simulink model "automata_learning"  (R2022a)
settings: Solver=FixedStepAuto  StartTime=0.0  StopTime=10.0  FixedStep=0.01  RelTol=1e-3
settings Model: Creator=diego  LastModifiedBy=diego

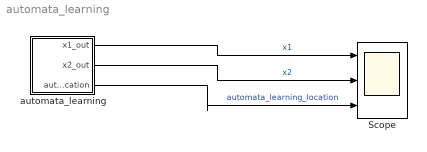
== system automata_learning ==
  Scope : Scope  NumInputPorts=3
  automata_learning : Stateflow chart  TreatAsAtomicUnit=on
  wires:
  automata_learning/1(x1_out) -> Scope/1  "x1"
  automata_learning/2(x2_out) -> Scope/2  "x2"
  automata_learning/3(automata_learning_location) -> Scope/3  "automata_learning_location"

== stateflow chart automata_learning/automata_learning ==
  settings: updateMethod=CONTINUOUS
  state loc1
    du:
    x1_dot = 17709872814793.0 * x2 / 147573952589676410000.0 - 4885549301075.0 * x1 / 295147905179352830000.0 - 25560522869469.0 * x1 * x2 / 36893488147419103000.0 + 23348987725423.0 * x1 ^ 2.0 / 295147905179352830000.0 + 37317396741413.0 * x2 ^ 2.0 / 36893488147419103000.0 + 0.9999999961747696;
    x2_dot = 4503599648254823.0 * x1 / 4503599627370496.0 + 475678987389.0 * x2 / 9223372036854776000.0 - 192670781808847.0 * x1 * x2 / 295147905179352830000.0 + 55569792035993.0 * x1 ^ 2.0 / 1180591620717411300000.0 + 336092630055397.0 * x2 ^ 2.0 / 295147905179352830000.0 - 0.0000000020426695939894023;
    x1_out=x1;
    x2_out=x2;
    automata_learning_location =1;
  state loc2
    du:
    x1_dot = 11278941379.0 * x1 * x2 / 2251799813685248.0 - 614502682225.0 * x2 / 36028797018963968.0 - 1617979564213.0 * x1 / 144115188075855872.0 + 2104648728409.0 * x1 ^ 2.0 / 1152921504606846980.0 - 9007161403513265.0 * x2 ^ 2.0 / 9007199254740992.0 + 0.00001782211096618136;
    x2_dot = 2069062415.0 * x1 / 1125899906842624.0 + 14700152253.0 * x2 / 4503599627370496.0 - 238660367459.0 * x1 * x2 / 288230376151711740.0 - 399866766279.0 * x1 ^ 2.0 / 1152921504606846980.0 - 55380855441.0 * x2 ^ 2.0 / 72057594037927936.0 - 1.0000030969954306;
    x1_out=x1;
    x2_out=x2;
    automata_learning_location =2;
  loc1 -> loc2 : [0.0009391 * x2 - 0.4996 * x1 + 1.0 < 0.0]
  (default) -> loc1 : {x1 = 0.0;
      | x2 = 0.0;}
  loc2 -> loc1 : [0.01034 * x1 + 196.7 * x2 + 1.0 < 0.0]
  data: x1_out output; x1 local; x2_out output; x2 local; automata_learning_location output
  data x1 settings: updateMethod=SF_CONTINUOUS_TIME_DATA
  data x2 settings: updateMethod=SF_CONTINUOUS_TIME_DATA
